simulink library "FirEven"  (R2022b)
settings: Solver=VariableStepAuto  StartTime=0.0  StopTime=10.0  RelTol=1e-3
undefined symbols (not defined in the file or in its folder): Row
libraries: HandyTextFile x6, TuneVar x3, FeaturePath x2, RTC x1, $bdroot x1, TOP x1
settings Model: Creator=jb10849  LastModifiedBy=fz1054048
settings SolverCC: AlgebraicLoopSolver=TrustRegion
settings DebuggingCC: UnconnectedInputMsg=warning  UnconnectedOutputMsg=warning  UnconnectedLineMsg=warning  SFMachineParentedDataDiag=warning  ArithmeticOperatorsInVariantConditions=warning
settings ModelReferenceCC: EnableRefExpFcnMdlSchedulingChecks=on
settings SFSimCC: SimUseLocalCustomCode=off  CustomCodeUndefinedFunction=UseInterfaceOnly
settings RTWCC: RTWUseLocalCustomCode=off  DLArmComputeVersion=19.05
settings CodeAppCC: StateflowObjectComments=on

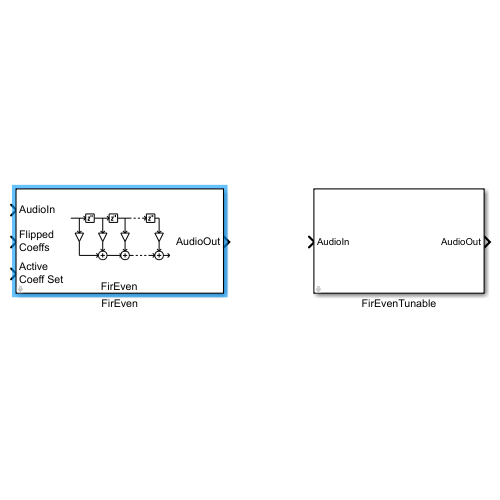
[thumbnail: Simulink's stored preview of the top-level diagram]
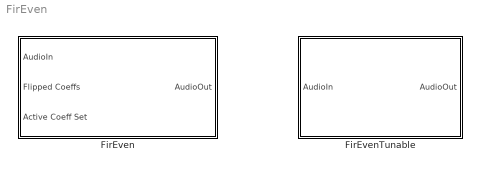
== system FirEven ==
  FirEven : Subsystem  mask(Blocklib FirEven){Config=[], FeatureName=FirEven}
      mask prompts: Config "FirEvenConfig"; FeatureName "Feature path name:"
      mask init:
      | blkh=gcbh;
      | Config=BTConfig.Assert(blkh,Config);
      | 
      | Config.Validate();
      | Config.DoMaskInit(blkh);
      mask TypeOptions FeatureName: FeaturePath/FeatureName
      mask Display:
      | [path,w,h] = IconFIR_Mask();
      | 
      | port_label('input', 1, 'AudioIn');
      | port_label('input', 2, sprintf('Flipped\nCoeffs'));
      | port_label('input', 3, sprintf('Active\nCoeff Set'));
      | port_label('output', 1, 'AudioOut');
      | 
      | % work in pixels since the icon does not scale
      | pos = get(gcbh,'position');
      | bw = pos(3) - pos(1);
      | bh = pos(4) - pos(2);
      | 
      | % Draw centered icon
      | xAdj = bw/2 - w/2;
      | yAdj = bh/2 - h/2 + 4;
      | for i=1:length(path)
      | %     patch(path(i).x+xAdj, path(i).y+yAdj, path(i).rgb);
      |     plot(path(i).x+xAdj, path(i).y+yAdj);
      | end
      | 
      | % Anchor the corners of the coordinate system
      | patch(0,0,[1 1 1]);
      | patch(bw,bh,[1 1 1]);
      | 
      | % Display some text
      | text(bw/2, 1,'FirEven', ...
      |     'horizontalAlignment','center', ...
      |     'VerticalAlignment','bottom');
  FirEvenTunable : Subsystem  mask(Blocklib FirEvenTunable){Config=[], FeatureName=FirEvenTunable}
      mask prompts: Config "FirEvenTunableConfig"; FeatureName "Feature path name:"
      mask init:
      | blkh=gcbh;
      | Config=BTConfig.Assert(blkh,Config);
      | 
      | Config.Validate();
      | Config.DoMaskInit(blkh);
      mask TypeOptions FeatureName: FeaturePath/FeatureName

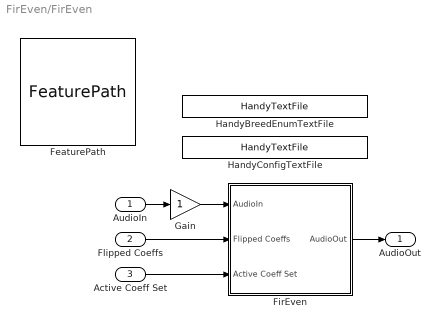
== system FirEven/FirEven ==
  AudioIn : Inport
  Flipped Coeffs : Inport  Port=2
  Active Coeff Set : Inport  Port=3
  FeaturePath : FeaturePath/FeaturePath  FeatureName=FirEven  IsGroup=off  GroupNumber=-1  IsModule=off  TriggerInit=[-5 -36 110 71]
      settings: SourceProductName=Bose Talaria
  FirEven : Subsystem  Variant=on
  Gain : Gain
  HandyBreedEnumTextFile : HandyTextFile/HandyTextFile  TemplateSource=<dialog fields>  FileSuffix=BreedEnum  OpenDialogOnLoad=off  UseThisBlockName=off  AddGrandParentNamePrefix=off  TheDefaultText=% $(FILENAME) $(PREFIX) $(SUFFIX)  ShowInLibBrowser=on
      settings: SourceProductName=Bose Talaria
  HandyConfigTextFile : HandyTextFile/HandyTextFile  TemplateSource=Config  FileSuffix=File  OpenDialogOnLoad=off  UseThisBlockName=off  AddGrandParentNamePrefix=off  TheDefaultText=% $(FILENAME) $(PREFIX) $(SUFFIX)  ShowInLibBrowser=on
      settings: SourceProductName=Bose Talaria
  AudioOut : Outport
  wires:
  AudioIn/1 -> Gain/1
  FirEven/1(AudioOut) -> AudioOut/1
  Flipped Coeffs/1 -> FirEven/2(Flipped Coeffs)
  Active Coeff Set/1 -> FirEven/3(Active Coeff Set)
  Gain/1 -> FirEven/1(AudioIn)

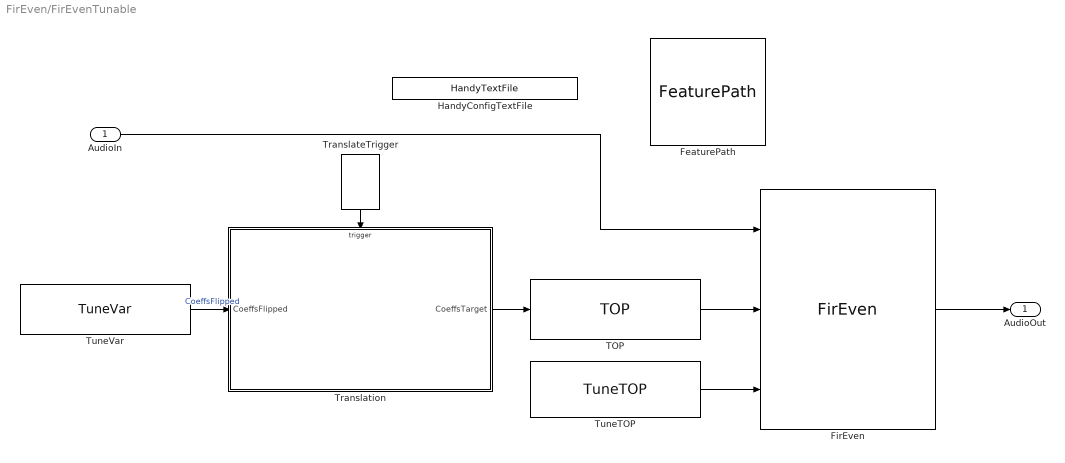
== system FirEven/FirEvenTunable ==
  AudioIn : Inport
  FeaturePath : FeaturePath/FeaturePath  FeatureName=FirEvenTunable  IsGroup=off  GroupNumber=-1  IsModule=off  TriggerInit=[235 -26 350 81]
      settings: SourceProductName=Bose Talaria
  FirEven : $bdroot/FirEven  Config=Config  FeatureName=FirEven
  HandyConfigTextFile : HandyTextFile/HandyTextFile  TemplateSource=Config  FileSuffix=File  OpenDialogOnLoad=off  UseThisBlockName=off  AddGrandParentNamePrefix=off  TheDefaultText=% $(FILENAME) $(PREFIX) $(SUFFIX)  ShowInLibBrowser=on
      settings: SourceProductName=Bose Talaria
  TOP : TOP/TOP  TriggerInit=[115 215 285 275]  TopName=CoeffsTarget  DataTypeOut=single  BankNumber=0  PreOverlay=false  PostOverlay=Config.PostOverlayRequired  CompatibilityString=Config.Breed  Role=Automatic
      settings: SourceProductName=Bose Talaria
  TranslateTrigger : TuneVar/TranslateTrigger  TriggerInit=[-74 90 -36 145]
      settings: SourceProductName=Bose Talaria
  Translation : MATLAB Function  TreatAsAtomicUnit=on  mask{Breed=Config.Breed, FrameSize=Config.FrameSize, MaxAvgCoeffLength=Config.MaxAvgCoeffLength, MaxNumFilters=Config.MaxNumFilters}
  TuneTOP : TuneVar/TuneTOP  TriggerInit=[115 297 285 353]  TopName=ActiveCoeffSet  TuneName=ActiveCoeffSet  DataTypeOut=uint32  TunabilityNumber=1  MinValue=[]  MaxValue=[]  BankNumber=0  PreOverlay=false  PostOverlay=Config.PostOverlayRequired  UseSameName=on  MaskValue=Config.TuneVarActiveCoeffSet
      settings: SourceProductName=Bose Talaria
  TuneVar : TuneVar/TuneVar  TuneName=CoeffsFlipped  SpecifyMaxSize=on  VariableDim=1 (Row)  MaxSize=[Config.MaxAvgCoeffLength, Config.MaxNumFilters]  TunabilityNumber=1  MinValue=[]  MaxValue=[]  TriggerInit=[-395 220 -225 270]  MaskValue=Config.TuneVarFirEvenCoeffsFlipped
      settings: SourceProductName=Bose Talaria
  AudioOut : Outport
  wires:
  AudioIn/1 -> FirEven/1
  FirEven/1 -> AudioOut/1
  TranslateTrigger/1 -> Translation/Trigger
  Translation/1(CoeffsTarget) -> TOP/1
  TuneVar/1 -> Translation/1(CoeffsFlipped)  "CoeffsFlipped"
  TOP/1 -> FirEven/2
  TuneTOP/1 -> FirEven/3

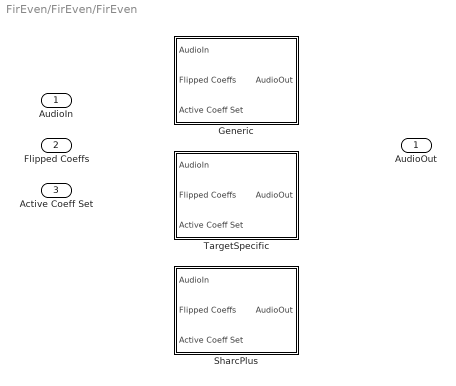
== system FirEven/FirEven/FirEven ==
  AudioIn : Inport
  Flipped Coeffs : Inport  Port=2
  Active Coeff Set : Inport  Port=3
  Generic : Subsystem  VariantControl=(default)
  SharcPlus : Subsystem  VariantControl=Config.Breed == AsdHwEnum.SharcPlus
  TargetSpecific : Subsystem  VariantControl=(Config.Breed == AsdHwEnum.Hexagon) || (Config.Breed == AsdHwEnum.ArmNeonV7V8)
  AudioOut : Outport

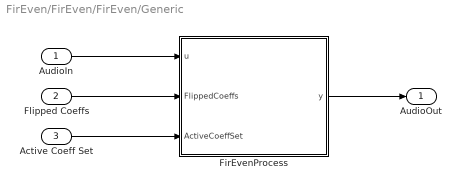
== system FirEven/FirEven/FirEven/Generic ==
  AudioIn : Inport
  Flipped Coeffs : Inport  Port=2
  Active Coeff Set : Inport  Port=3
  FirEvenProcess : MATLAB Function  TreatAsAtomicUnit=on
  AudioOut : Outport
  wires:
  FirEvenProcess/1(y) -> AudioOut/1
  Flipped Coeffs/1 -> FirEvenProcess/2(FlippedCoeffs)
  AudioIn/1 -> FirEvenProcess/1(u)
  Active Coeff Set/1 -> FirEvenProcess/3(ActiveCoeffSet)

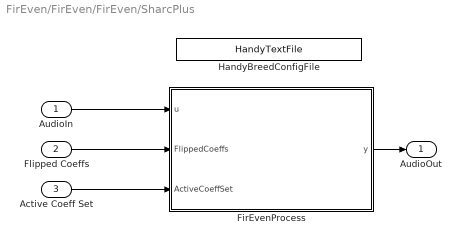
== system FirEven/FirEven/FirEven/SharcPlus ==
  AudioIn : Inport
  Flipped Coeffs : Inport  Port=2
  Active Coeff Set : Inport  Port=3
  FirEvenProcess : MATLAB Function  TreatAsAtomicUnit=on
  HandyBreedConfigFile : HandyTextFile/HandyTextFile  TemplateSource=<dialog fields>  FileSuffix=BreedConfig  OpenDialogOnLoad=off  UseThisBlockName=off  AddGrandParentNamePrefix=on  TheDefaultText=|  ShowInLibBrowser=on
      | % $(FILENAME) Setup model parameters for each "Init" callback (e.g. update diagram)
      | sample_rate_in_hertz = 44100;
      | frame_size = 32;
      | sysin_channel_count = 2;
      settings: SourceProductName=Bose Talaria
  AudioOut : Outport
  wires:
  FirEvenProcess/1(y) -> AudioOut/1
  Active Coeff Set/1 -> FirEvenProcess/3(ActiveCoeffSet)
  Flipped Coeffs/1 -> FirEvenProcess/2(FlippedCoeffs)
  AudioIn/1 -> FirEvenProcess/1(u)

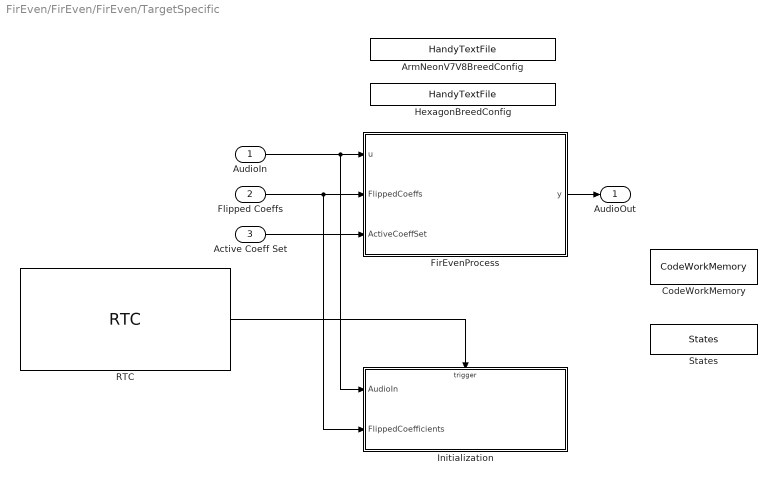
== system FirEven/FirEven/FirEven/TargetSpecific ==
  AudioIn : Inport
  Flipped Coeffs : Inport  Port=2
  Active Coeff Set : Inport  Port=3
  ArmNeonV7V8BreedConfig : HandyTextFile/HandyTextFile  TemplateSource=<dialog fields>  FileSuffix=File  OpenDialogOnLoad=off  UseThisBlockName=on  AddGrandParentNamePrefix=on  TheDefaultText=|  ShowInLibBrowser=on
      | % $(FILENAME) Setup model parameters for each "Init" callback (e.g. update diagram)
      | sample_rate_in_hertz = 44100;
      | frame_size = 32;
      | sysin_channel_count = 2;
      settings: SourceProductName=Bose Talaria
  CodeWorkMemory : DataStoreMemory  DataStoreName=CodeWorkMemory  WriteAfterWriteMsg=warning  InitialValue=uint32(zeros(1,17+4*Config.BreedObj.MaxNumOfThreads+14*Config.BreedObj.MaxNumOfThreads))  ShowAdditionalParam=off  OutDataTypeStr=uint32
  FirEvenProcess : MATLAB Function  TreatAsAtomicUnit=on  mask{Breed=Config.Breed}
  HexagonBreedConfig : HandyTextFile/HandyTextFile  TemplateSource=<dialog fields>  FileSuffix=File  OpenDialogOnLoad=off  UseThisBlockName=on  AddGrandParentNamePrefix=on  TheDefaultText=|  ShowInLibBrowser=on
      | % $(FILENAME) Setup model parameters for each "Init" callback (e.g. update diagram)
      | sample_rate_in_hertz = 44100;
      | frame_size = 32;
      | sysin_channel_count = 2;
      settings: SourceProductName=Bose Talaria
  Initialization : Subsystem
  RTC : RTC/RTC  REQ_Priority=RTC_Mask.NormalPriority  RequestAtInit=on  EnableRequest=on  REQElemType1=uint32  REQElemWidth1=1  REQElemInitial1=[]  REQElemType2=uint32  REQElemWidth2=1  REQElemInitial2=[]  REQElemType3=uint32  REQElemWidth3=1  REQElemInitial3=[]  REQElemType4=uint32  REQElemWidth4=1  REQElemInitial4=[]  REQElemType5=uint32  REQElemWidth5=1  REQElemInitial5=[]  REQElemType6=uint32  REQElemWidth6=1  REQElemInitial6=[]  REQElemType7=uint32  REQElemWidth7=1  REQElemInitial7=[]  REQElemType8=uint32  REQElemWidth8=1  REQElemInitial8=[]  REQElemType9=uint32  REQElemWidth9=1  REQElemInitial9=[]  REQElemType10=uint32  REQElemWidth10=1  REQElemInitial10=[]  EnableResponse=off  EnableRSP_StatusIn=off  RSPElemType1=uint32  RSPElemWidth1=1  RSPElemType2=uint32  RSPElemWidth2=1  RSPElemType3=uint32  RSPElemWidth3=1  RSPElemType4=uint32  RSPElemWidth4=1  RSPElemType5=uint32  RSPElemWidth5=1  RSPElemType6=uint32  RSPElemWidth6=1  RSPElemType7=uint32  RSPElemWidth7=1  RSPElemType8=uint32  RSPElemWidth8=1  RSPElemType9=uint32  RSPElemWidth9=1  RSPElemType10=uint32  RSPElemWidth10=1  EnableNotification=off  EnableNTF_PrepTrig=off  NTFElemType1=uint32  NTFElemWidth1=1  NTFElemType2=uint32  NTFElemWidth2=1  NTFElemType3=uint32  NTFElemWidth3=1  NTFElemType4=uint32  NTFElemWidth4=1  NTFElemType5=uint32  NTFElemWidth5=1  NTFElemType6=uint32  NTFElemWidth6=1  NTFElemType7=uint32  NTFElemWidth7=1  NTFElemType8=uint32  NTFElemWidth8=1  NTFElemType9=uint32  NTFElemWidth9=1  NTFElemType10=uint32  NTFElemWidth10=1  MaskMessageName=InitReset
      settings: SourceProductName=Bose Talaria
  States : DataStoreMemory  DataStoreName=States  WriteAfterWriteMsg=warning  InitialValue=single(zeros(Config.BreedObj.StateBufferSize,1))  ShowAdditionalParam=off  OutDataTypeStr=single
  AudioOut : Outport
  wires:
  AudioIn/1 -> Initialization/1(AudioIn), FirEvenProcess/1(u)
  Flipped Coeffs/1 -> Initialization/2(FlippedCoefficients), FirEvenProcess/2(FlippedCoeffs)
  Active Coeff Set/1 -> FirEvenProcess/3(ActiveCoeffSet)
  FirEvenProcess/1(y) -> AudioOut/1
  RTC/1 -> Initialization/Trigger

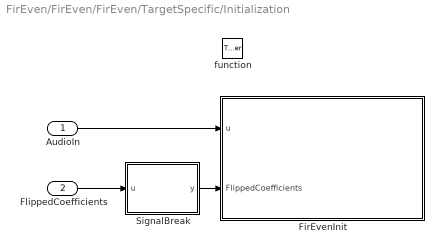
== system FirEven/FirEven/FirEven/TargetSpecific/Initialization ==
  AudioIn : Inport
  FlippedCoefficients : Inport  Port=2
  function : TriggerPort  TriggerType=function-call  VariantControl=(inherit)
  FirEvenInit : MATLAB Function  TreatAsAtomicUnit=on  mask{MaxNumOfThreds=Config.BreedObj.MaxNumOfThreads, MaxAvgCoeffLength=Config.MaxAvgCoeffLength, Breed=Config.Breed}
  SignalBreak : MATLAB Function  TreatAsAtomicUnit=on
  wires:
  SignalBreak/1(y) -> FirEvenInit/2(FlippedCoefficients)
  FlippedCoefficients/1 -> SignalBreak/1(u)
  AudioIn/1 -> FirEvenInit/1(u)

== matlab function FirEven/FirEven/TargetSpecific/Initialization/SignalBreak ==
  data: u input; y output
function y = fcn(u)

y = u;
end

== matlab function FirEven/FirEven/Generic/FirEvenProcess ==
  data: u input; FlippedCoeffs input; y output; ActiveCoeffSet input
function y = FirEvenProcess(u, FlippedCoeffs, ActiveCoeffSet)

[~, NumChannels] = size(u);

y = FirEvenProcessSim(u, NumChannels, ActiveCoeffSet, FlippedCoeffs);

end



% % Extract configuration information from inputs
% [taps, ~] = size(flipped_coeffs);
% [frame_size, num_channels] = size(u);
% 
% % Initialize state variables to zero
% persistent states;
% if isempty(states)
%     states = single(zeros(taps + 2, num_channels));
% end
% % Initialize state index to zero
% persistent state_index;
% if isempty(state_index)
%     state_index = uint32(0);
% end
% 
% % Set correct data types
% filter_length = uint32(taps);
% frame_size = uint32(frame_size);
% num_channels = uint32(num_channels);
% active_coeff_set = uint32(active_coeff_set);
% % Invoking the fir_even function
% y = fir_even(u, frame_size, num_channels, states, filter_length, state_index, active_coeff_set, flipped_coeffs);
% 
% 
% function y = fir_even(u, framesize, numChannels, states, filterLength, stateIndex, activeCoeffSet, coeffs)
% % If target == codegen, generate warning if no CRL found
% coder.replace('-warnifnoreplacement');
% 
% % If running simulation, just use filter()
% % Matlab function takes unflipped coeffs, so coeffs needs to be flipped
% a = 1;
% b = flipud(coeffs);
% [taps, ~] = size(b);
% 
% persistent zi;
% if isempty(zi)
%     zi = single(zeros(taps - 1, numChannels));
% end
% 
% y = single(zeros(size(u)));
% for i = 1:numChannels
%     % Get input, filter coeffs and state for this channel
%     u0 = u(:, i);
%     filterIdx = activeCoeffSet(i) + 1; % add 1 for Matlab indexing
%     coeff = b(:, filterIdx);
%     state = zi(:, i);
%     
%     % Compute output samples and state
%     [y0, state] = filter(coeff, a, u0, state);
%     y(:, i) = y0;
%     
%     % Save state
%     zi(:, i) = state;
% end

== matlab function FirEven/FirEven/TargetSpecific/Initialization/FirEvenInit ==
  data: u input; FlippedCoefficients input; CodeWorkMemory data_store_memory; MaxNumOfThreds parameter; MaxAvgCoeffLength parameter; Breed parameter
function FirEvenInit(u, FlippedCoefficients, MaxNumOfThreds, MaxAvgCoeffLength, Breed)

% Extract configuration information from inputs
[FilterLength, NumFilters] = size(FlippedCoefficients);
[FrameSize, NumChannels] = size(u);


% Error if MaxAvgCoeffLength is less than than Filters passed into the
% block
if MaxAvgCoeffLength < FilterLength
    error("Coefficients of length [%d] supplied through signal ports should have length less than or equal to [MaxAvgCoeffLength] property of value %d.", FilterLength, MaxAvgCoeffLength);
end

% Zero Padd Coeffs to front to make coeffs to be length [MaxAvgCoeffLength] 
FlippedCoefficients = [zeros(MaxAvgCoeffLength - FilterLength,NumFilters,class(FlippedCoefficients)); FlippedCoefficients];

global CodeWorkMemory;

% Simulation 
if(coder.target('MATLAB') || coder.target('Sfun')) 
    return; % No init for simulation code
else
    switch(Breed)
        case(AsdHwEnum.Hexagon)
            y = fireven_hexagon_init(uint32(FrameSize), uint32(NumChannels), uint32(NumFilters), uint32(MaxAvgCoeffLength), single(FlippedCoefficients), uint32(CodeWorkMemory), uint32(MaxNumOfThreds));
            % NOTE: The CRL mechanism requires an output for the function call,
            % and appears to be optimized out if that return value isn't used. 
            % This is a dummy operation to make sure CRL ends up in generated code
            CodeWorkMemory(1) = y;
        case(AsdHwEnum.ArmNeonV7V8)
            y = fireven_armv7v8_process_init(uint32(FrameSize), uint32(NumChannels), uint32(NumFilters), uint32(MaxAvgCoeffLength), single(FlippedCoefficients), uint32(CodeWorkMemory));
            % NOTE: The CRL mechanism requires an output for the function call,
            % and appears to be optimized out if that return value isn't used. 
            % This is a dummy operation to make sure CRL ends up in generated code
            CodeWorkMemory(1) = y;
    end
end
end

function y = fireven_hexagon_init(frame_size, num_ch, num_of_filters, filter_len, FlippedCoefficients, workMemory, maxNumOfThreds)
coder.replace('-errorifnoreplacement');
[taps, ~] = size(FlippedCoefficients);
y=frame_size + num_ch + num_of_filters + filter_len + taps + workMemory(1);
end
function y = fireven_armv7v8_process_init(frame_size, num_ch, num_of_filters, filter_len, FlippedCoefficients, workMemory)
coder.replace('-errorifnoreplacement');
[taps, ~] = size(FlippedCoefficients);
y=frame_size + num_ch + num_of_filters + filter_len + taps + workMemory(1);
end

== matlab function FirEven/FirEven/TargetSpecific/FirEvenProcess ==
  data: u input; y output; FlippedCoeffs input; ActiveCoeffSet input; CodeWorkMemory data_store_memory; States data_store_memory; Breed parameter
function y = FirEvenProcess(u, FlippedCoeffs, ActiveCoeffSet, Breed)

% Extract configuration information from inputs
[FilterLength, ~] = size(FlippedCoeffs);
[FrameSize, NumChannels] = size(u);

global CodeWorkMemory;
global States;
 
% Initialize variables
% persistent States;
% if isempty(States)
%     States = single(zeros(FilterLength + FrameSize*2 + 2, NumChannels));
% end

% Set correct data types
FilterLength = uint32(FilterLength);
FrameSize = uint32(FrameSize);
ActiveCoeffSet = uint32(ActiveCoeffSet);


if(coder.target('MATLAB') || coder.target('Sfun')) 
    % FIREVEN SIMULATION
    y = FirEvenProcessSim(u, NumChannels, ActiveCoeffSet, FlippedCoeffs);
else
    switch(Breed)
        case(AsdHwEnum.Hexagon)
            % FIR EVEN HEXAGON
            if (FilterLength > FrameSize)
                y = fireven_hexagon_process_mt(single(u), uint32(ActiveCoeffSet), single(States), uint32(CodeWorkMemory));
            else
                y = fireven_hexagon_process_lt(single(u), uint32(ActiveCoeffSet), single(States), uint32(CodeWorkMemory));
            end
        case(AsdHwEnum.ArmNeonV7V8)
            % FIR EVEN ARM
            y = fireven_armv7v8_process(single(u), uint32(ActiveCoeffSet), single(States), uint32(CodeWorkMemory));
    end
end    
end
  

function y = fireven_hexagon_process_mt(u, ActiveCoeffSet, States, WorkMemory)
coder.replace('-errorifnoreplacement');
[fs, num_ch]  = size(u);
y = single(zeros(fs, num_ch));
end

function y = fireven_hexagon_process_lt(u, ActiveCoeffSet, States, WorkMemory)
coder.replace('-errorifnoreplacement');
[fs, num_ch]  = size(u);
y = single(zeros(fs, num_ch));
end

function y = fireven_armv7v8_process(u, ActiveCoeffSet, States, WorkMemory)
coder.replace('-errorifnoreplacement');
[fs, num_ch]  = size(u);
y = single(zeros(fs, num_ch));
end

== matlab function FirEven/FirEvenTunable/Translation ==
  data: CoeffsFlipped input; CoeffsTarget output; Breed parameter; FrameSize parameter; MaxAvgCoeffLength parameter; MaxNumFilters parameter
  events: trigger input FUNCTION_CALL_EVENT
function CoeffsTarget  = FirEvenTranslationMfb(CoeffsFlipped, Breed, FrameSize, MaxAvgCoeffLength, MaxNumFilters)
IsCoeffsRawFlipped = true;                          % Assume Coefficients are already flipped

% Check that CoeffsFlipped is appropriately sized.
if CoeffsFlipped.Size(1) > MaxAvgCoeffLength
    TranslateError('Length of CoeffsFlipped must not be greater than MaxAvgCoeffLength');
end

if not(CoeffsFlipped.Size(2) <= MaxNumFilters)
    TranslateError('Number of Filters in CoeffsFlipped must be less than or equal to MaxNumFilters');
end

CoeffsFlippedValue = CoeffsFlipped.Value;

CoeffsRaw = zeros(MaxAvgCoeffLength, MaxNumFilters, class(CoeffsFlippedValue));
CoeffsRaw(MaxAvgCoeffLength - CoeffsFlipped.Size(1) + 1 : MaxAvgCoeffLength, 1:CoeffsFlipped.Size(2)) = CoeffsFlippedValue;

[CoeffsTarget] = FirEvenTranslation(CoeffsRaw, Breed, MaxNumFilters, MaxAvgCoeffLength, FrameSize, IsCoeffsRawFlipped);


end

== matlab function FirEven/FirEven/SharcPlus/FirEvenProcess ==
  data: u input; y output; FlippedCoeffs input; ActiveCoeffSet input
function y = FirEvenProcess(u, FlippedCoeffs, ActiveCoeffSet)

% Extract configuration information from inputs
[FilterLength, ~] = size(FlippedCoeffs);
[FrameSize, NumChannels] = size(u);

% Initialize variables
persistent States;
if isempty(States)
    States = single(zeros(FilterLength + FrameSize + 2, NumChannels));
end

% Initialize state index to zero
persistent StateIndex;
if isempty(StateIndex)
    StateIndex = uint32(0);
end


if(coder.target('MATLAB') || coder.target('Sfun')) 
    % FIREVEN SIMULATION
    y = FirEvenProcessSim(u, NumChannels, ActiveCoeffSet, FlippedCoeffs);
else
    y = fir_even(single(u), uint32(FrameSize), uint32(NumChannels), single(States), ...
        uint32(FilterLength), uint32(StateIndex), uint32(ActiveCoeffSet), single(FlippedCoeffs));
end

end

function y = fir_even(u, FrameSize, NumChannels, States, FilterLength, StateIndex, ActiveCoeffSet, Coeffs)
% If target == codegen, generate warning if no CRL found
coder.replace('-warnifnoreplacement');
y = single(zeros(FrameSize, NumChannels));
end
